simulink model "RDA_EMG_FES"  (R2020b)
settings: Solver=VariableStepAuto  StartTime=0.0  StopTime=100000  RelTol=1e-3
undefined symbols (not defined in the file or in its folder): f
libraries: dspnetwork x4, sldrtlib x1, instrumentlib x1
settings Model: Creator=ayurkewi  LastModifiedBy=Wacom hrg
settings DataIOCC: ReturnWorkspaceOutputs=off
settings DebuggingCC: ArithmeticOperatorsInVariantConditions=warning
settings SFSimCC: CustomCodeUndefinedFunction=UseInterfaceOnly

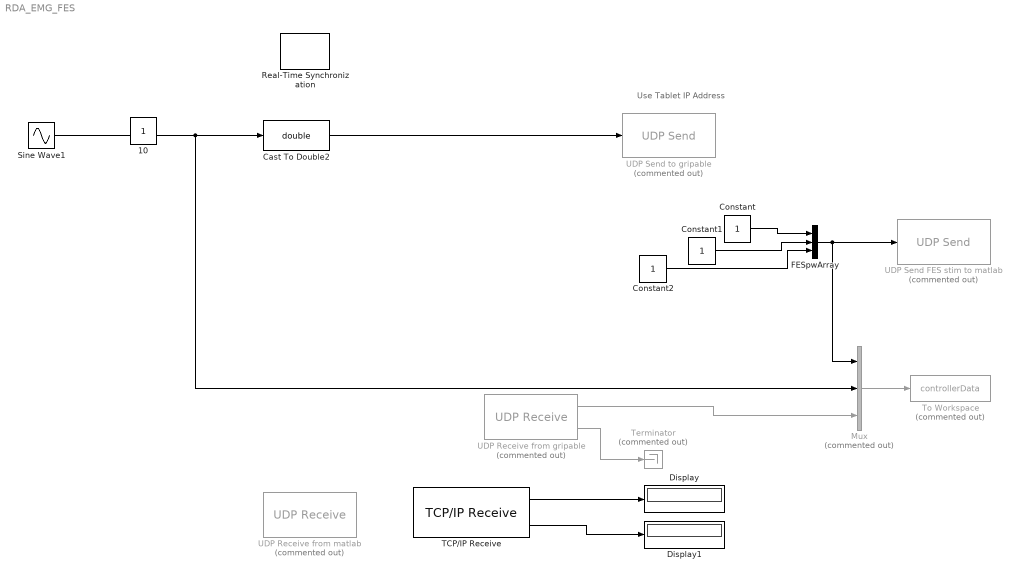
== system RDA_EMG_FES ==
  note: Use Tablet IP Address
  Cast To Double2 : DataTypeConversion  OutDataTypeStr=double
  Constant : Constant
  Constant1 : Constant
  Constant2 : Constant
  Display : Display
  Display1 : Display
  FESpwArray : Mux  Inputs=3
  Mux : Mux  Commented=on  Inputs=3
  Real-Time Synchronization : sldrtlib/Real-Time Synchronization  SampleTime=0.001  MaxMissedTicks=100000  ShowMissedTicks=off  YieldWhenWaiting=off
  Sine Wave1 : Sin  Amplitude=0.015  Bias=0.025  Frequency=0.1  Phase=3/2 *pi  SampleTime=0
  TCP/IP Receive : instrumentlib/TCP//IP Receive  Host="\"localhost\""  Port=4002  DataSize=1  EnableBlockingMode=off  Timeout=10  SampleTime=0.01  DataType=double  ByteOrder=BigEndian  ASCIIFormatting=%f,  Terminator=LF
  Terminator : Terminator  Commented=on
  To Workspace : ToWorkspace  Commented=on  VariableName=controllerData  SaveFormat=Timeseries  SampleTime=0.02
  UDP Receive from gripable : dspnetwork/UDP Receive  Commented=on  localURL='0.0.0.0'  localPort=26000  remoteURL='0.0.0.0'  remotePort=-1  recvBufferSize=1024  dims=1  signalDatatype=double  isComplex=off  isVarSize=off  showBlockingTime=off  blockingTime=0  sampletime=0.02  blockPlatform=[]
  UDP Receive from matlab : dspnetwork/UDP Receive  Commented=on  localURL='0.0.0.0'  localPort=5000  remoteURL='0.0.0.0'  remotePort=-1  recvBufferSize=1024  dims=1  signalDatatype=double  isComplex=off  isVarSize=off  showBlockingTime=off  blockingTime=0  sampletime=0.001  blockPlatform=[]
  UDP Send FES stim to matlab : dspnetwork/UDP Send  Commented=on  remoteURL='127.0.0.1'  remotePort=22392  localURL='0.0.0.0'  localPortSource=Automatically determine  localPort=-1  sendBufferSize=8190  sampletime=-1  blockPlatform=[]  separateLengthPort=0
  UDP Send to gripable : dspnetwork/UDP Send  Commented=on  remoteURL='146.169.203.41'  remotePort=25000  localURL='0.0.0.0'  localPortSource=Automatically determine  localPort=-1  sendBufferSize=8192  sampletime=-1  blockPlatform=[]  separateLengthPort=0
  10 : Constant  IOType=siggen
  wires:
  Cast To Double2/1 -> UDP Send to gripable/1
  Sine Wave1/1 -> Mux/2, Cast To Double2/1
  FESpwArray/1 -> Mux/1, UDP Send FES stim to matlab/1
  UDP Receive from gripable/2 -> Terminator/1
  UDP Receive from gripable/1 -> Mux/3
  Mux/1 -> To Workspace/1
  Constant/1 -> FESpwArray/1
  Constant1/1 -> FESpwArray/2
  Constant2/1 -> FESpwArray/3
  TCP/IP Receive/1 -> Display/1
  TCP/IP Receive/2 -> Display1/1
